simulink model "train_val_model"  (R2021a)
settings: Solver=VariableStepAuto  StartTime=0.0  StopTime=10.0  RelTol=1e-3
libraries: simulink x2, pid_lib x2
settings Model: Creator=hty  LastModifiedBy=hty

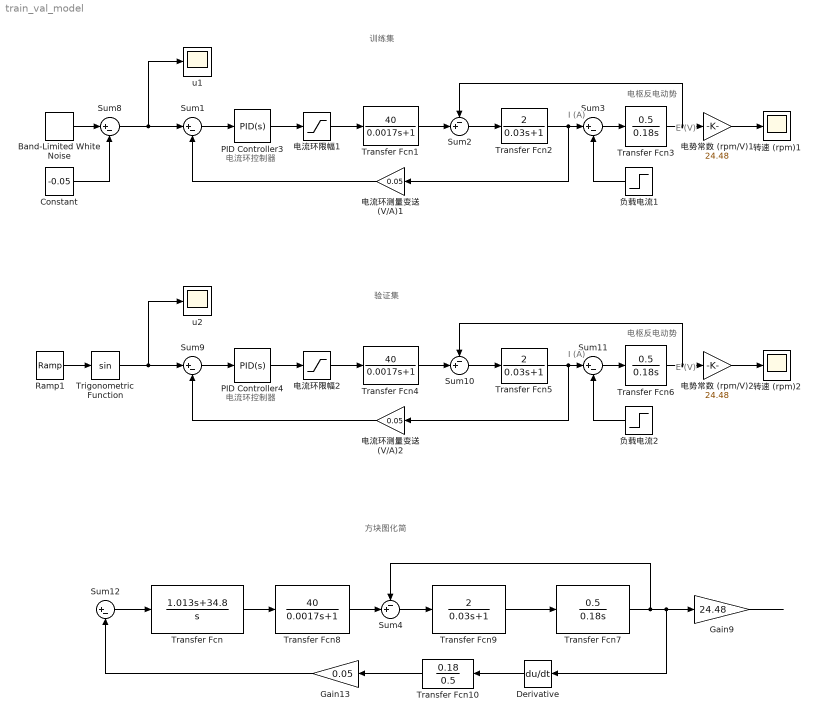
== system train_val_model ==
  note: 方块图化简
  note: 训练集
  note: 电枢反电动势
  note: I (A)
  note: I (A)
  note: 电流环控制器
  note: E (V)
  note: 电流环控制器
  note: E (V)
  note: 电枢反电动势
  note: 验证集
  Band-Limited White Noise : simulink/Sources/Band-Limited White Noise  Cov=[0.001]  Ts=0.001  seed=[23341]
  Constant : Constant  Value=-0.05
  Derivative : Derivative
  Gain13 : Gain  Gain=0.05
  Gain9 : Gain  Gain=24.48
  PID Controller3 : pid_lib/PID Controller  Controller=PID  Form=Parallel  TimeDomain=Continuous-time  UseExternalTs=off  SampleTime=-1  IntegratorMethod=Forward Euler  FilterMethod=Forward Euler  ControllerParametersSource=internal  P=1.013  I=34.8  D=0  UseFilter=on  N=100  TunerSelectOption=Transfer Function Based (PID Tuner App)  InitialConditionSource=internal  InitialConditionForIntegrator=0  InitialConditionForFilter=0  DifferentiatorICPrevScaledInput=0  ExternalReset=none  TrackingMode=off  Kt=1  LimitOutput=off  SatLimitsSource=internal  UpperSaturationLimit=inf  LowerSaturationLimit=-inf  LinearizeAsGain=on  AntiWindupMode=none  Kb=1  POutMin=[]  POutMax=[]  IOutMin=[]  IOutMax=[]  DOutMin=[]  DOutMax=[]  NOutMin=[]  NOutMax=[]  SumOutMin=[]  SumOutMax=[]  SaturationOutMin=[]  SaturationOutMax=[]  PParamMin=[]  PParamMax=[]  IParamMin=[]  IParamMax=[]  DParamMin=[]  DParamMax=[]  NParamMin=[]  NParamMax=[]  KbParamMin=[]  KbParamMax=[]  KtParamMin=[]  KtParamMax=[]  KbOutMin=[]  KbOutMax=[]  KtOutMin=[]  KtOutMax=[]  IntegratorOutMin=[]  IntegratorOutMax=[]  FilterOutMin=[]  FilterOutMax=[]  SumI1OutMin=[]  SumI1OutMax=[]  SumI2OutMin=[]  SumI2OutMax=[]  SumI3OutMin=[]  SumI3OutMax=[]  SumI4OutMin=[]  SumI4OutMax=[]  SumDOutMin=[]  SumDOutMax=[]  DifferentiatorOutMin=[]  DifferentiatorOutMax=[]  FilterDiffOutCoefMin=[]  FilterDiffOutCoefMax=[]  ReciprocalOutMin=[]  ReciprocalOutMax=[]  SumDenOutMin=[]  SumDenOutMax=[]  SumNumOutMin=[]  SumNumOutMax=[]  DivideOutMin=[]  DivideOutMax=[]  UdiffTsProdOutMin=[]  UdiffTsProdOutMax=[]  NTsProdOutMin=[]  NTsProdOutMax=[]  UintegralTsProdOutMin=[]  UintegralTsProdOutMax=[]  UngainTsProdOutMin=[]  UngainTsProdOutMax=[]  IntegratorContinuousStateAttributes=''  IntegratorStateMustResolveToSignalObject=off  IntegratorRTWStateStorageClass=Auto  FilterContinuousStateAttributes=''  FilterStateMustResolveToSignalObject=off  FilterRTWStateStorageClass=Auto  ParallelPVariant=InternalParameters  IdealPVariant=Disabled  IVariant=InternalParameters  DVariant=InternalParameters  IntegratorVariant=Continuous  SatVariant=Disabled  AWVariant=Passthrough  PCopyVariant=Disabled  TRVariant=Disabled  FdbkBlocksVariant=Forward  IdealPFdbkVariant=Disabled  SatFdbkVariant=Disabled  DerivativeFilterVariant=ContFilter  NVariant=InternalParameters  NCopyVariant=Disabled  FilterICVariant=InternalICsFilter  IntegratorICVariant=InternalICs  ExternalResetVariant=Disabled  TRSumVariant=Passthrough  SumFdbkVariant=Disabled  SumVariant=Sum_PID  TsampFilterVariant=InternalTs  TsampNgainVariant=Passthrough  TsampIntegralVariant=Passthrough  ExternalSaturationOutDataTypeStr=Inherit: Same as second input
  PID Controller4 : pid_lib/PID Controller  Controller=PID  Form=Parallel  TimeDomain=Continuous-time  UseExternalTs=off  SampleTime=-1  IntegratorMethod=Forward Euler  FilterMethod=Forward Euler  ControllerParametersSource=internal  P=1.013  I=34.8  D=0  UseFilter=on  N=100  TunerSelectOption=Transfer Function Based (PID Tuner App)  InitialConditionSource=internal  InitialConditionForIntegrator=0  InitialConditionForFilter=0  DifferentiatorICPrevScaledInput=0  ExternalReset=none  TrackingMode=off  Kt=1  LimitOutput=off  SatLimitsSource=internal  UpperSaturationLimit=inf  LowerSaturationLimit=-inf  LinearizeAsGain=on  AntiWindupMode=none  Kb=1  POutMin=[]  POutMax=[]  IOutMin=[]  IOutMax=[]  DOutMin=[]  DOutMax=[]  NOutMin=[]  NOutMax=[]  SumOutMin=[]  SumOutMax=[]  SaturationOutMin=[]  SaturationOutMax=[]  PParamMin=[]  PParamMax=[]  IParamMin=[]  IParamMax=[]  DParamMin=[]  DParamMax=[]  NParamMin=[]  NParamMax=[]  KbParamMin=[]  KbParamMax=[]  KtParamMin=[]  KtParamMax=[]  KbOutMin=[]  KbOutMax=[]  KtOutMin=[]  KtOutMax=[]  IntegratorOutMin=[]  IntegratorOutMax=[]  FilterOutMin=[]  FilterOutMax=[]  SumI1OutMin=[]  SumI1OutMax=[]  SumI2OutMin=[]  SumI2OutMax=[]  SumI3OutMin=[]  SumI3OutMax=[]  SumI4OutMin=[]  SumI4OutMax=[]  SumDOutMin=[]  SumDOutMax=[]  DifferentiatorOutMin=[]  DifferentiatorOutMax=[]  FilterDiffOutCoefMin=[]  FilterDiffOutCoefMax=[]  ReciprocalOutMin=[]  ReciprocalOutMax=[]  SumDenOutMin=[]  SumDenOutMax=[]  SumNumOutMin=[]  SumNumOutMax=[]  DivideOutMin=[]  DivideOutMax=[]  UdiffTsProdOutMin=[]  UdiffTsProdOutMax=[]  NTsProdOutMin=[]  NTsProdOutMax=[]  UintegralTsProdOutMin=[]  UintegralTsProdOutMax=[]  UngainTsProdOutMin=[]  UngainTsProdOutMax=[]  IntegratorContinuousStateAttributes=''  IntegratorStateMustResolveToSignalObject=off  IntegratorRTWStateStorageClass=Auto  FilterContinuousStateAttributes=''  FilterStateMustResolveToSignalObject=off  FilterRTWStateStorageClass=Auto  ParallelPVariant=InternalParameters  IdealPVariant=Disabled  IVariant=InternalParameters  DVariant=InternalParameters  IntegratorVariant=Continuous  SatVariant=Disabled  AWVariant=Passthrough  PCopyVariant=Disabled  TRVariant=Disabled  FdbkBlocksVariant=Forward  IdealPFdbkVariant=Disabled  SatFdbkVariant=Disabled  DerivativeFilterVariant=ContFilter  NVariant=InternalParameters  NCopyVariant=Disabled  FilterICVariant=InternalICsFilter  IntegratorICVariant=InternalICs  ExternalResetVariant=Disabled  TRSumVariant=Passthrough  SumFdbkVariant=Disabled  SumVariant=Sum_PID  TsampFilterVariant=InternalTs  TsampNgainVariant=Passthrough  TsampIntegralVariant=Passthrough  ExternalSaturationOutDataTypeStr=Inherit: Same as second input
  Ramp1 : simulink/Sources/Ramp  slope=5  start=0  InitialOutput=0
  Sum{1,3,8..9,11..12} (6 alike) : Sum  Inputs=|+-
  Sum10 : Sum  Inputs=-+|
  Sum2 : Sum  Inputs=-+|
  Sum4 : Sum  Inputs=-+|
  Transfer Fcn : TransferFcn  Numerator=[1.013 34.8]  Denominator=[1 0]
  Transfer Fcn1 : TransferFcn  Numerator=40  Denominator=[0.0017 1]
  Transfer Fcn10 : TransferFcn  Numerator=0.18  Denominator=[0.5]
  Transfer Fcn2 : TransferFcn  Numerator=2  Denominator=[0.03 1]
  Transfer Fcn3 : TransferFcn  Numerator=0.5  Denominator=[0.18 0]
  Transfer Fcn4 : TransferFcn  Numerator=40  Denominator=[0.0017 1]
  Transfer Fcn5 : TransferFcn  Numerator=2  Denominator=[0.03 1]
  Transfer Fcn6 : TransferFcn  Numerator=0.5  Denominator=[0.18 0]
  Transfer Fcn7 : TransferFcn  Numerator=0.5  Denominator=[0.18 0]
  Transfer Fcn8 : TransferFcn  Numerator=40  Denominator=[0.0017 1]
  Transfer Fcn9 : TransferFcn  Numerator=2  Denominator=[0.03 1]
  Trigonometric Function : Trigonometry
  u1 : Scope
  u2 : Scope
  电势常数 (rpm/V)1 : Gain  Gain=24.48
  电势常数 (rpm/V)2 : Gain  Gain=24.48
  电流环测量变送 (V/A)1 : Gain  Gain=0.05
  电流环测量变送 (V/A)2 : Gain  Gain=0.05
  电流环限幅1 : Saturate  UpperLimit=50  LowerLimit=-50
  电流环限幅2 : Saturate  UpperLimit=50  LowerLimit=-50
  负载电流1 : Step  Time=3  After=0  SampleTime=0
  负载电流2 : Step  Time=3  After=0  SampleTime=0
  转速 (rpm)1 : Scope
  转速 (rpm)2 : Scope
  wires:
  电流环测量变送 (V/A)1/1 -> Sum1/2
  电流环测量变送 (V/A)2/1 -> Sum9/2
  PID Controller4/1 -> 电流环限幅2/1
  Trigonometric Function/1 -> u2/1, Sum9/1
  电流环限幅1/1 -> Transfer Fcn1/1
  Transfer Fcn2/1 -> 电流环测量变送 (V/A)1/1, Sum3/1
  电势常数 (rpm/V)2/1 -> 转速 (rpm)2/1
  Sum2/1 -> Transfer Fcn2/1
  Sum11/1 -> Transfer Fcn6/1
  负载电流1/1 -> Sum3/2
  Sum9/1 -> PID Controller4/1
  Transfer Fcn5/1 -> 电流环测量变送 (V/A)2/1, Sum11/1
  Transfer Fcn4/1 -> Sum10/2
  电势常数 (rpm/V)1/1 -> 转速 (rpm)1/1
  Transfer Fcn1/1 -> Sum2/2
  Sum1/1 -> PID Controller3/1
  PID Controller3/1 -> 电流环限幅1/1
  Sum8/1 -> u1/1, Sum1/1
  Sum10/1 -> Transfer Fcn5/1
  Transfer Fcn3/1 -> Sum2/1, 电势常数 (rpm/V)1/1
  Transfer Fcn6/1 -> Sum10/1, 电势常数 (rpm/V)2/1
  Sum3/1 -> Transfer Fcn3/1
  负载电流2/1 -> Sum11/2
  电流环限幅2/1 -> Transfer Fcn4/1
  Constant/1 -> Sum8/2
  Band-Limited White Noise/1 -> Sum8/1
  Ramp1/1 -> Trigonometric Function/1
  Derivative/1 -> Transfer Fcn10/1
  ? -> Sum12/1
  Transfer Fcn8/1 -> Sum4/2
  Transfer Fcn9/1 -> Transfer Fcn7/1
  Transfer Fcn10/1 -> Gain13/1
  Sum4/1 -> Transfer Fcn9/1
  Transfer Fcn/1 -> Transfer Fcn8/1
  Transfer Fcn7/1 -> Derivative/1, Gain9/1, Sum4/1
  Sum12/1 -> Transfer Fcn/1
  Gain13/1 -> Sum12/2
  Gain9/1 -> ?
